simulink model "Controllers_Complete"  (R2021b)
settings: Solver=FixedStepAuto  StartTime=0  StopTime=20  FixedStep=0.002  RelTol=1e-3  EnableMultiTasking=on
PostLoadFcn:
  | qc_set_target_type(getConfigSet(bdroot, 'QUARC Default Target Configuration'));
values from neighbouring files (symbols this model uses):
  k = place(sysest_cont.A, sysest_cont.B, new_pole)    [Recursive.m]
  K_lqr = lqr(sysest_cont,Q,R)    [Recursive.m]
  K_p = 1/K_dc(1)    [AdaptivePPLvl2.m]
  K_pp = place(A, B, new_pole)    [AdaptivePPLvl2.m]
  Kr = 1/Kdc(1)    [Recursive.m]
  L_obs = place(sysest_cont.A',sysest_cont.C',1.5*new_pole)'    [Recursive.m]
  param = [disc(1).Numerator{:}(3:end) -disc(1).Denominator{:}(2:end)]    [Recursive.m]
  param2 = [disc(2).Numerator{:}(3:end) -disc(2).Denominator{:}(2:end)]    [Recursive.m]
  sysest_ct = sysest_cont    [Recursive.m]
  Trans = block.InputPort(1).Data    [AdaptivePPLvl2.m]
  Ts = 0.002    [AdaptivePPLvl2.m]
  v_a_max = 5    [Recursive.m]
undefined symbols (not defined in the file or in its folder): DiscIntNeverNeededParam, HIL, k2, K_lqr_eta, K_lqr_x, K_pp_en_eta, K_pp_en_x, Kr2, L22, L_KF, magnitude, Q_KF, qc_get_step_size, R_KF, sigbuilder_block, sysest, sysfake_ct
libraries: simulink_extras x7, ctrlSharedLib x4, quarc_library x4, cstblocks x1
settings Model: SimulationMode=external  ExtModeTrigDuration=5000  Creator=CFulford  LastModifiedBy=jesuc
settings SolverCC: AlgebraicLoopSolver=TrustRegion  PositivePriorityOrder=on
settings DataIOCC: LimitDataPoints=on  SaveFormat=Array  SignalLoggingSaveFormat=ModelDataLogs  ReturnWorkspaceOutputs=off
settings OptimizationCC: ExpressionDepthLimit=2147483647  InitFltsAndDblsToZero=on  LifeSpan=inf
settings DebuggingCC: SaveWithParameterizedLinksMsg=none  UnderspecifiedInitializationDetection=Classic  MergeDetectMultiDrivingBlocksExec=none  SolverPrmCheckMsg=warning  MultiTaskDSMMsg=warning  MultiTaskCondExecSysMsg=none  FcnCallInpInsideContextMsg=warning  StateNameClashWarn=warning  SFUnexpectedBacktrackingDiag=warning  SFNoUnconditionalDefaultTransitionDiag=warning  SFExecutionAtInitializationDiag=none  SFMachineParentedDataDiag=warning  ArithmeticOperatorsInVariantConditions=warning
settings HardwareCC: ProdBitPerPointer=32  ProdBitPerSizeT=32  ProdBitPerPtrDiffT=32  ProdLargestAtomicFloat=None  ProdIntDivRoundTo=Undefined  ProdEndianess=Unspecified  ProdWordSize=32  ProdHWDeviceType=32-bit Generic
settings ModelReferenceCC: PropagateSignalLabelsOutOfModel=off
settings SFSimCC: SimUseLocalCustomCode=off  CustomCodeUndefinedFunction=UseInterfaceOnly
settings RTWCC: Description=QUARC Win64 Target  SystemTargetFile=quarc_win64.tlc  TemplateMakefile=quarc_default_tmf  RTWUseLocalCustomCode=off
settings CodeAppCC: StateflowObjectComments=on
settings STFCustomTargetCC: TargetPreCompLibLocation=C:\PROGRA~3\QUARC\lib\2019b\win64\release  ConcurrentExecutionCompliant=on  CombineOutputUpdateFcns=on  CPPClassGenCompliant=on  GRTInterface=off  SystemTargetFile=quarc_win64.tlc
settings GRTTargetCC: TargetPreCompLibLocation=C:\PROGRA~3\QUARC\lib\2019b\win64\release  TargetLangStandard=C89/C90 (ANSI)  ParMdlRefBuildCompliant=off  CompOptLevelCompliant=off  MatFileLogging=off  UseToolchainInfoCompliant=off  ExtMode=on  ExtModeMexFile=quarc_comm
settings ConfigComp: CovMetricSettings=dw  CovSaveCumulativeToWorkspaceVar=on  CovSaveSingleToWorkspaceVar=on  CovExternalEMLEnable=off  CovSFcnEnable=off

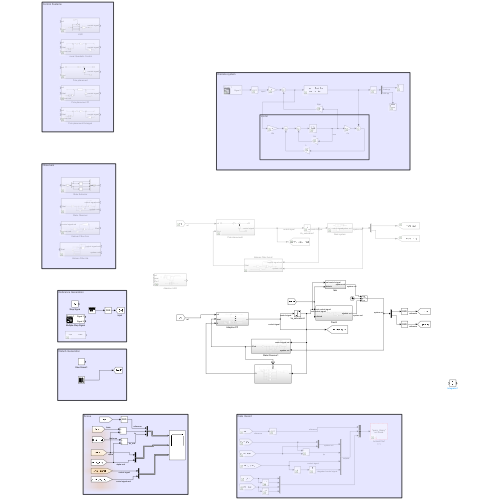
[thumbnail: Simulink's stored preview of the top-level diagram]
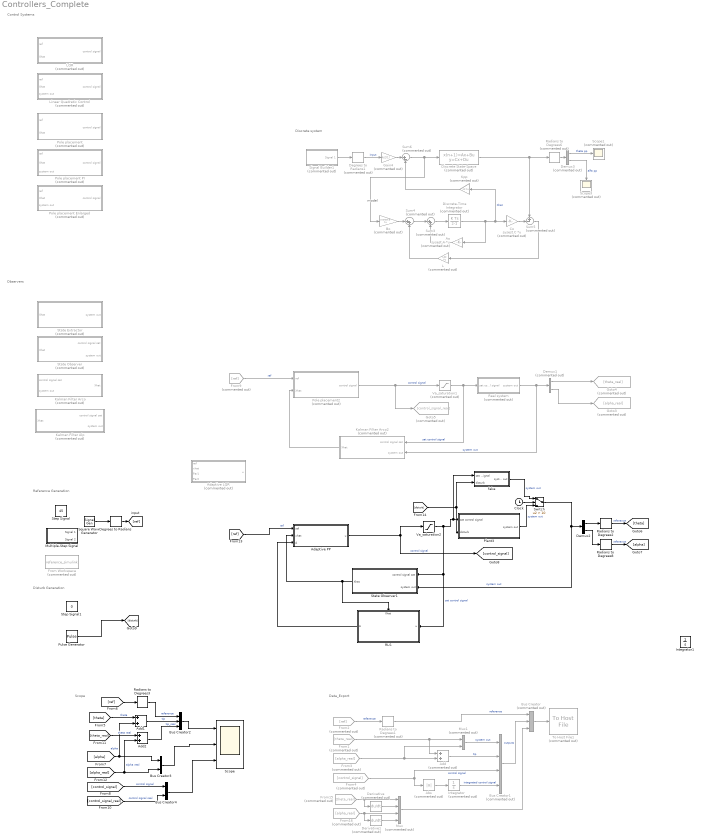
== system Controllers_Complete ==
  note: Reference Generation
  note: Disturb Generation
  note: Data_Export
  note: Scope
  note: Control Systems
  note: Observers
  note: Discrete system
  note: model
  Abs : Abs  Commented=on
  Adaptive LQR : Subsystem  Commented=on
  Adaptive PP : Subsystem
  Add : Sum  Commented=on
  Add1 : Sum
  Add2 : Sum
  Ao : Gain  Commented=on  Gain=sysest.A  Multiplication=Matrix(K*u)
  Bo : Gain  Commented=on  Gain=sysest.B  Multiplication=Matrix(K*u)
  Bus Creator : BusCreator  Commented=on  Inputs=3
  Bus Creator1 : BusCreator  Commented=on  Inputs=4
  Bus Creator2 : BusCreator  Inputs=3
  Bus Creator3 : BusCreator  Inputs=2
  Bus Creator4 : BusCreator  Inputs=2
  Clock : Clock
  Co : Gain  Commented=on  Gain=sysest.C  Multiplication=Matrix(K*u)
  Degrees to Radians : simulink_extras/Transformations/Degrees to Radians
  Degrees to Radians1 : simulink_extras/Transformations/Degrees to Radians  Commented=on
  Demux1 : Demux  Commented=on  Outputs=2
  Demux2 : Demux  Outputs=2
  Demux3 : Demux  Commented=on  Outputs=2
  Derivative : Derivative  Commented=on
  Derivative1 : Derivative  Commented=on
  Discrete State-Space : DiscreteStateSpace  Commented=on  A=sysest.A  B=sysest.B  C=sysest.C  D=sysest.D  SampleTime=0.002
  Discrete-Time Integrator : DiscreteIntegrator  Commented=on  SampleTime=0.002  ICPrevOutput=DiscIntNeverNeededParam  ICPrevScaledInput=DiscIntNeverNeededParam
  From Workspace : FromWorkspace  Commented=on  VariableName=reference_simulink
  From1 : From  Commented=on  GotoTag=theta_real
  From15 : From  Commented=on  GotoTag=theta_real
  From16 : From  Commented=on  GotoTag=alpha_real
  From2 : From  Commented=on  GotoTag=ref
  From3 : From  Commented=on  GotoTag=alpha_real
  From4 : From  Commented=on  GotoTag=control_signal
  From9 : From  Commented=on  GotoTag=ref
  Gain4 : Gain  Commented=on  Gain=Kr2(1)
  Goto3 : Goto  Commented=on  GotoTag=alpha_real
  Goto4 : Goto  Commented=on  GotoTag=theta_real
  Goto5 : Goto  Commented=on  GotoTag=control_signal_real
  Integrator : Integrator  Commented=on
  Integrator1 : Integrator
  Kalman Filter Alp : Subsystem  Commented=on
  Kalman Filter Arco : Subsystem  Commented=on
  Kalman Filter Arco2 : Subsystem  Commented=on
  Kpp : Gain  Commented=on  Gain=k2  Multiplication=Matrix(K*u)
  L : Gain  Commented=on  Gain=L22  Multiplication=Matrix(K*u)
  LQR : Subsystem  Commented=on
  Linear Quadratic Control : Subsystem  Commented=on
  Multiple-Step Signal : Subsystem  Tag=STV Subsys  LoadFcn=sigbuilder_block('load');  StartFcn=sigbuilder_block('start');  StopFcn=sigbuilder_block('stop');  ClipboardFcn=sigbuilder_block('clipboard');  mask(Sigbuilder block){tuvar=[0:10]}
      mask help: Simulink:masks:SigbuilderBlock_MD
      mask init:
      | if ~strcmp(get_param(bdroot(gcbh),'SimulationStatus'),'stopped') tuvar = sigbuilder_block('maskInit'); end
      settings: CopyFcn=sigbuilder_block('copy');  DeleteFcn=sigbuilder_block('delete');  ModelCloseFcn=sigbuilder_block('modelClose');  PreSaveFcn=sigbuilder_block('preSave');  PauseFcn=sigbuilder_block('pause');  ContinueFcn=sigbuilder_block('continue');  NameChangeFcn=sigbuilder_block('namechange');  OpenFcn=sigbuilder_block('open',[5.4 5.4 1141.2 580.8 ]);  CloseFcn=sigbuilder_block('close');
      mask Display: plot(0, 0, 100, 100,[2, 2, 32, 32, 2], [68, 8, 8, 68, 68],[32, 2], [38, 38], [32, 19, 2],[53, 60, 44], [32, 17, 17, 2],[16, 16, 31, 31]);txt = getActiveGroup(gcbh);text(2, 100, txt,'verticalAlignment', 'top');
  Mux : Mux  Commented=on
  Mux1 : Mux  Commented=on  Inputs=2
  Plant3 : Subsystem
  Pole placement : Subsystem  Commented=on
  Pole placement Enlarged : Subsystem  Commented=on
  Pole placement PI : Subsystem  Commented=on
  Pole placement2 : Subsystem  Commented=on
  Pulse Generator : DiscretePulseGenerator  PulseType=Time based  Amplitude=0.001  Period=1  PulseWidth=50
  RLS : Subsystem
      settings: PortSchema="{\"entries\":[{\"content\":{\"sides\":[{\"content\":{\"connectorIds\":[\"In1\"]},\"type\":\"ConnectorPlacement.EquallySpacedRectSide\",\"uuid\":\"553c4a9d-f21a-4a66-a87a-a243cd55d2e3\"},{\"content\":{\"connectorIds\":[\"Out1\"],\"side\":\"RIGHT\"},\"type\":\"ConnectorPlacement.EquallySpacedRectSide\",\"uuid\":\"7c0c7ce9-5483-43cc-b177-6c3304c50a8e\"},{\"content\":{\"connectorIds\":[\"In2\"],\"side\":\"TOP\"},\"type\":\"ConnectorPlacement.EquallySpacedRectSide\",\"uuid\":\"5face929-888d-4c99-9f40-f5add7f5ece6\"}]},\"type\":\"ConnectorPlacement.EquallySpacedConnector\",\"uuid\":\"9b2ed38d-f553-46ca-b742-367219c23a2d\"}],\"packageUris\":[\"http://schema.mathworks.com/mf0/Connector/R2020b\"],\"version\":\"1.0\"}"
  Radians to Degrees1 : simulink_extras/Transformations/Radians to Degrees  Commented=on
  Radians to Degrees2 : simulink_extras/Transformations/Radians to Degrees
  Radians to Degrees3 : simulink_extras/Transformations/Radians to Degrees
  Radians to Degrees6 : simulink_extras/Transformations/Radians to Degrees  Commented=on
  Radians to Degrees8 : simulink_extras/Transformations/Radians to Degrees
  Real system : Subsystem  Commented=on
  Scope : Scope  NumInputPorts=3
  Scope1 : Scope  Commented=on
  Scope3 : Scope  Commented=on
  Signal Builder1 : Subsystem  Tag=STV Subsys  Commented=on  LoadFcn=sigbuilder_block('load');  StartFcn=sigbuilder_block('start');  StopFcn=sigbuilder_block('stop');  ClipboardFcn=sigbuilder_block('clipboard');  mask(Sigbuilder block){tuvar=[0:10]}
      mask help: Simulink:masks:SigbuilderBlock_MD
      mask init:
      | if ~strcmp(get_param(bdroot(gcbh),'SimulationStatus'),'stopped') tuvar = sigbuilder_block('maskInit'); end
      settings: CopyFcn=sigbuilder_block('copy');  DeleteFcn=sigbuilder_block('delete');  ModelCloseFcn=sigbuilder_block('modelClose');  PreSaveFcn=sigbuilder_block('preSave');  PauseFcn=sigbuilder_block('pause');  ContinueFcn=sigbuilder_block('continue');  NameChangeFcn=sigbuilder_block('namechange');  OpenFcn=sigbuilder_block('open',[437.6 199.2 550.4 400 ]);  CloseFcn=sigbuilder_block('close');
      mask Display: plot(0, 0, 100, 100,[2, 2, 32, 32, 2], [68, 8, 8, 68, 68],[32, 2], [38, 38], [32, 19, 2],[53, 60, 44], [32, 17, 17, 2],[16, 16, 31, 31]);txt = getActiveGroup(gcbh);text(2, 100, txt,'verticalAlignment', 'top');
  Square Wave Generator : SignalGenerator  WaveForm=square  Amplitude=45  Frequency=3  Units=rad/sec
  State Extractor : Subsystem  Commented=on
  State Observer : Subsystem  Commented=on
  State Observer1 : Subsystem
  Step Signal : Constant  Value=45
  Step Signal1 : Constant  Value=0
  Sum3 : Sum  Commented=on  Inputs=|++
  Sum4 : Sum  Commented=on  Inputs=|++
  Sum5 : Sum  Commented=on  Inputs=+-|
  Sum6 : Sum  Commented=on  Inputs=|+-
  Switch : Switch  Criteria=u2 > Threshold  Threshold=10
  To Host File1 : quarc_library/Sinks/To Host/To Host File  Commented=on  file_name=Sine tests\Sine_24_in_theta_alpha.mat  variable_name=data  decimation=1  sample_time=-1  file_format=MAT-file v.4  options=No header or footer  append=off  final_file_name=Sine tests\Sine_24_in_theta_alpha.mat  bitrate=2000000
  Va_saturation1 : Saturate  Commented=on  UpperLimit=v_a_max  LowerLimit=-v_a_max
  Va_saturation2 : Saturate  UpperLimit=v_a_max  LowerLimit=-v_a_max
  fake : Subsystem
  wires:
  Bus Creator2/1 -> Scope/1
  Bus Creator3/1 -> Scope/2
  Pole placement2/1(" control signal") -> Goto5/1, Va_saturation1/1  "control signal"
  From4/1 -> Abs/1, Bus Creator1/3  "control signal"
  Bus Creator1/1 -> Bus Creator/2  "outputs"
  [disturb] -> fake/2(disturb), Plant3/2(disturb)
  Demux2/1 -> Radians to Degrees2/1
  Adaptive PP/1(u) -> Va_saturation2/1, [control_signal]  "control signal"
  [ref] -> Adaptive PP/1(ref)  "ref"
  From1/1 -> Add/1, Mux1/1
  [control_signal_real] -> Bus Creator4/2  "control signal real"
  Add/1 -> Bus Creator1/2  "tip"
  From2/1 -> Radians to Degrees1/1  "reference"
  Integrator/1 -> Bus Creator1/4  "integrated control signal"
  Bus Creator/1 -> To Host File1/1
  [alpha_real] -> Bus Creator3/2, Add2/2  "alpha real"
  Demux1/1 -> Goto4/1
  Real system/1(system out) -> Kalman Filter Arco2/2(system out), Demux1/1  "system out"
  [theta_real] -> Add2/1  "theta real"
  Va_saturation2/1 -> State Observer1/1(control signal sat), RLS/1(u), Plant3/1(sat control signal), fake/1(sat control signal)  "sat control signal"
  From3/1 -> Add/2, Mux1/2
  Demux1/2 -> Goto3/1
  Switch/1 -> State Observer1/2(system out), Demux2/1  "system out"
  [control_signal] -> Bus Creator4/1  "control signal"
  Degrees to Radians/1 -> [ref]
  Bus Creator4/1 -> Scope/3
  Radians to Degrees3/1 -> Bus Creator2/1  "reference"
  Va_saturation1/1 -> Kalman Filter Arco2/1(control signal sat), Real system/1(sat control signal)  "sat control signal"
  [alpha] -> Bus Creator3/1, Add1/2  "alpha"
  Mux1/1 -> Bus Creator1/1  "system out"
  [theta] -> Add1/1  "theta"
  Demux2/2 -> Radians to Degrees8/1
  Sum5/1 -> L/1
  Demux3/1 -> Scope1/1  "theta pp"
  Sum6/1 -> Discrete State-Space/1, Bo/1
  L/1 -> Sum4/2
  Discrete State-Space/1 -> Radians to Degrees6/1, Sum5/1
  Sum4/1 -> Sum3/1
  Sum3/1 -> Discrete-Time Integrator/1
  Degrees to Radians1/1 -> Gain4/1  "input"
  Co/1 -> Sum5/2
  Demux3/2 -> Scope3/1  "alfa pp"
  Signal Builder1/1(Signal 1) -> Degrees to Radians1/1
  Kpp/1 -> Sum6/2
  Bo/1 -> Sum4/1
  Discrete-Time Integrator/1 -> Ao/1, Kpp/1, Co/1  "Xhat"
  Gain4/1 -> Sum6/1
  Ao/1 -> Sum3/2
  Radians to Degrees6/1 -> Demux3/1
  From9/1 -> Pole placement2/1(ref)  "ref"
  Add1/1 -> Bus Creator2/2  "tip"
  Add2/1 -> Bus Creator2/3  "tip_real"
  [ref] -> Radians to Degrees3/1
  Radians to Degrees1/1 -> Bus Creator/1  "reference"
  Radians to Degrees2/1 -> [theta]  "reference"
  Radians to Degrees8/1 -> [alpha]  "reference"
  State Observer1/1(Xhat) -> Adaptive PP/2(xhat), RLS/2(Xhat)
  Kalman Filter Arco2/1(Xhat) -> Pole placement2/2(Xhat)
  Abs/1 -> Integrator/1
  From15/1 -> Derivative/1, Mux/1
  From16/1 -> Derivative1/1, Mux/3
  Mux/1 -> Bus Creator/3
  Derivative/1 -> Mux/2
  Derivative1/1 -> Mux/4
  RLS/1(A) -> Adaptive PP/3(A)
  Pulse Generator/1 -> [disturb]
  fake/1(system out) -> Switch/1  "system out"
  Plant3/1(system out) -> Switch/3  "system out"
  Square Wave Generator/1 -> Degrees to Radians/1
  Clock/1 -> Switch/2

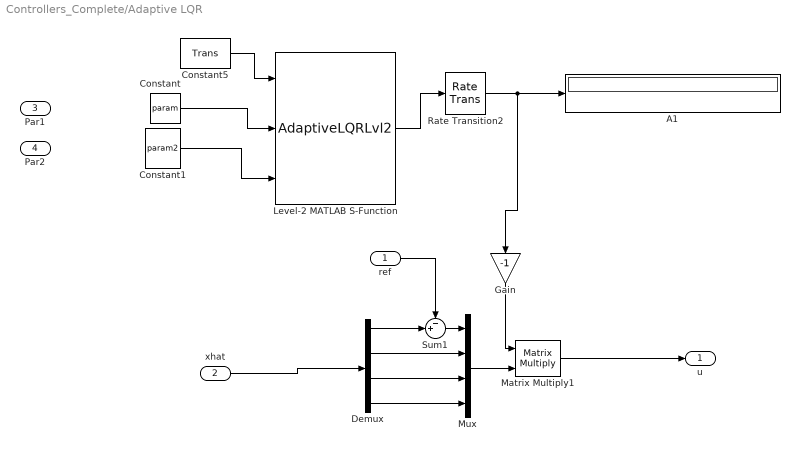
== system Controllers_Complete/Adaptive LQR ==
  ref : Inport
  xhat : Inport  Port=2
  Par1 : Inport  Port=3
  Par2 : Inport  Port=4
  A1 : Display
  Constant : Constant  Value=param
  Constant1 : Constant  Value=param2
  Constant5 : Constant  Value=Trans  SampleTime=Ts
  Demux : Demux
  Gain : Gain  Gain=-1
  Level-2 MATLAB S-Function : M-S-Function  FunctionName=AdaptiveLQRLvl2
  Matrix Multiply1 : Product  Multiplication=Matrix(*)
  Mux : Mux
  Rate Transition2 : RateTransition  InitialCondition=k
  Sum1 : Sum  Inputs=-+|
  u : Outport
  wires:
  Constant5/1 -> Level-2 MATLAB S-Function/1
  Constant/1 -> Level-2 MATLAB S-Function/2
  Level-2 MATLAB S-Function/1 -> Rate Transition2/1
  Rate Transition2/1 -> Gain/1, A1/1
  Constant1/1 -> Level-2 MATLAB S-Function/3
  ref/1 -> Sum1/1
  Sum1/1 -> Mux/1
  Demux/2 -> Mux/2
  Demux/4 -> Mux/4
  Demux/3 -> Mux/3
  Demux/1 -> Sum1/2
  xhat/1 -> Demux/1
  Matrix Multiply1/1 -> u/1
  Mux/1 -> Matrix Multiply1/2
  Gain/1 -> Matrix Multiply1/1

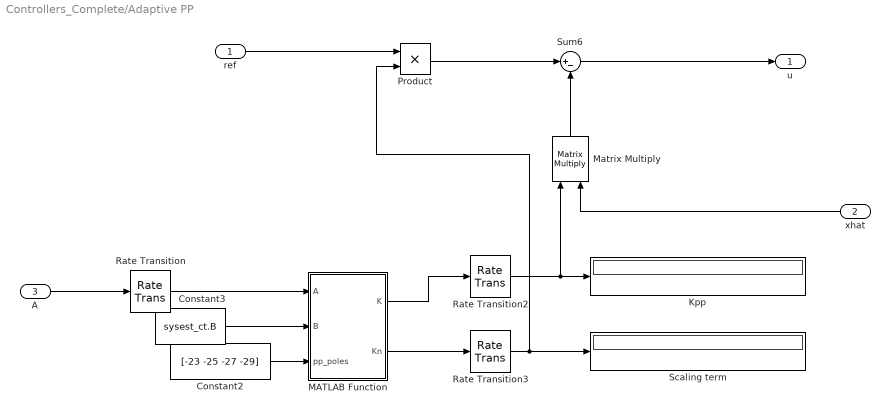
== system Controllers_Complete/Adaptive PP ==
  ref : Inport
  xhat : Inport  Port=2
  A : Inport  Port=3
  Constant2 : Constant  Value=[-23 -25 -27 -29]  SampleTime=0.2
  Constant3 : Constant  Value=sysest_ct.B  SampleTime=0.2
  Kpp : Display
  MATLAB Function : MATLAB Function  TreatAsAtomicUnit=on
  Matrix Multiply : Product  Multiplication=Matrix(*)
  Product : Product
  Rate Transition : RateTransition  InitialCondition=sysest_ct.A  OutPortSampleTime=0.2
  Rate Transition2 : RateTransition  InitialCondition=k
  Rate Transition3 : RateTransition  InitialCondition=Kr
  Scaling term : Display
  Sum6 : Sum  Inputs=|+-
  u : Outport
  wires:
  Product/1 -> Sum6/1
  Sum6/1 -> u/1
  Matrix Multiply/1 -> Sum6/2
  ref/1 -> Product/1
  MATLAB Function/2(Kn) -> Rate Transition3/1
  Rate Transition/1 -> MATLAB Function/1(A)
  MATLAB Function/1(K) -> Rate Transition2/1
  Rate Transition2/1 -> Kpp/1, Matrix Multiply/1
  Rate Transition3/1 -> Product/2, Scaling term/1
  xhat/1 -> Matrix Multiply/2
  A/1 -> Rate Transition/1
  Constant2/1 -> MATLAB Function/3(pp_poles)
  Constant3/1 -> MATLAB Function/2(B)

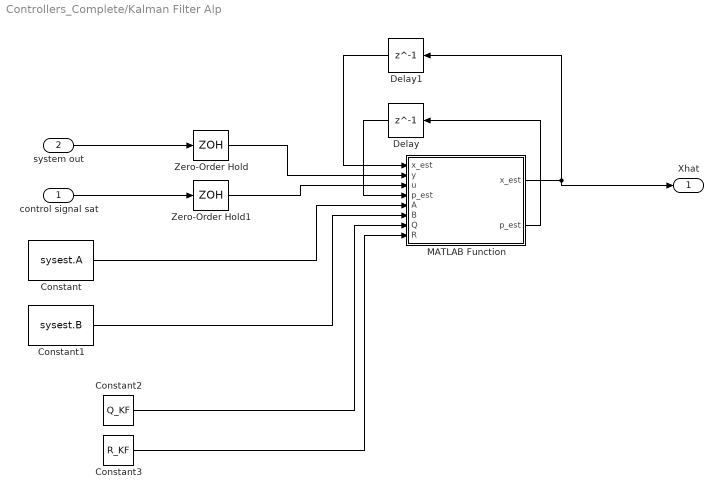
== system Controllers_Complete/Kalman Filter Alp ==
  control signal sat : Inport
  system out : Inport  Port=2
  Constant : Constant  Value=sysest.A
  Constant1 : Constant  Value=sysest.B
  Constant2 : Constant  Value=Q_KF
  Constant3 : Constant  Value=R_KF
  Delay : Delay  DelayLength=1  InitialCondition=eye(4)
  Delay1 : Delay  DelayLength=1  InitialCondition=[0;0;0;0]
  MATLAB Function : MATLAB Function  TreatAsAtomicUnit=on
  Zero-Order Hold : ZeroOrderHold  SampleTime=0.002
  Zero-Order Hold1 : ZeroOrderHold  SampleTime=0.002
  Xhat : Outport
  wires:
  MATLAB Function/1(x_est) -> Xhat/1, Delay1/1
  Delay/1 -> MATLAB Function/4("p_est ")
  MATLAB Function/2(p_est) -> Delay/1
  Zero-Order Hold1/1 -> MATLAB Function/3(u)
  Constant1/1 -> MATLAB Function/6(B)
  Delay1/1 -> MATLAB Function/1("x_est ")
  Constant/1 -> MATLAB Function/5(A)
  Zero-Order Hold/1 -> MATLAB Function/2(y)
  control signal sat/1 -> Zero-Order Hold1/1
  system out/1 -> Zero-Order Hold/1
  Constant2/1 -> MATLAB Function/7(Q)
  Constant3/1 -> MATLAB Function/8(R)

== system Controllers_Complete/Kalman Filter Arco ==
  control signal sat : Inport  PortDimensions=1
  system out : Inport  Port=2  PortDimensions=2
  Add : Sum  Inputs=+++
  Gain : Gain  Gain=sysest_ct.B  Multiplication=Matrix(K*u) (u vector)
  Gain1 : Gain  Gain=L_KF  Multiplication=Matrix(K*u) (u vector)
  Gain2 : Gain  Gain=sysest_ct.A - L_KF * sysest_ct.C  Multiplication=Matrix(K*u) (u vector)
  Integrator : Integrator
  Xhat : Outport  PortDimensions=4
  wires:
  Gain2/1 -> Add/1
  Integrator/1 -> Gain2/1, Xhat/1  "x_hat"
  Add/1 -> Integrator/1  "x_hat_dot"
  Gain/1 -> Add/2
  control signal sat/1 -> Gain/1
  Gain1/1 -> Add/3
  system out/1 -> Gain1/1

== system Controllers_Complete/Kalman Filter Arco2 ==
  control signal sat : Inport  PortDimensions=1
  system out : Inport  Port=2  PortDimensions=2
  Add : Sum  Inputs=+++
  Gain : Gain  Gain=sysest_ct.B  Multiplication=Matrix(K*u) (u vector)
  Gain1 : Gain  Gain=L_KF  Multiplication=Matrix(K*u) (u vector)
  Gain2 : Gain  Gain=sysest_ct.A - L_KF * sysest_ct.C  Multiplication=Matrix(K*u) (u vector)
  Integrator : Integrator
  Xhat : Outport  PortDimensions=4
  wires:
  Gain2/1 -> Add/1
  Integrator/1 -> Gain2/1, Xhat/1  "x_hat"
  Add/1 -> Integrator/1  "x_hat_dot"
  Gain/1 -> Add/2
  control signal sat/1 -> Gain/1
  Gain1/1 -> Add/3
  system out/1 -> Gain1/1

== system Controllers_Complete/LQR ==
  ref : Inport
  Xhat : Inport  Port=2
  Demux : Demux
  Gain3 : Gain  Gain=-K_lqr  Multiplication=Matrix(K*u)
  Mux : Mux
  Sum1 : Sum  Inputs=-+|
  " control signal" : Outport
  wires:
  ref/1 -> Sum1/1
  Xhat/1 -> Demux/1
  Demux/1 -> Sum1/2
  Demux/2 -> Mux/2
  Demux/3 -> Mux/3
  Demux/4 -> Mux/4
  Gain3/1 -> " control signal"/1
  Sum1/1 -> Mux/1
  Mux/1 -> Gain3/1

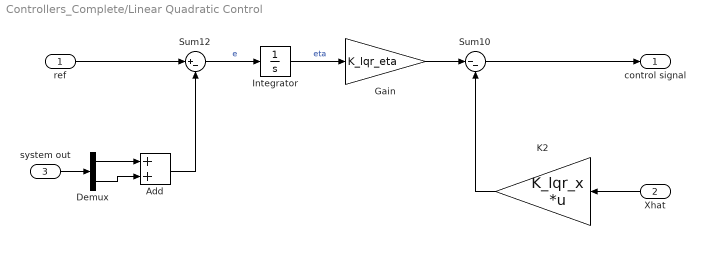
== system Controllers_Complete/Linear Quadratic Control ==
  ref : Inport
  Xhat : Inport  Port=2
  system out : Inport  Port=3
  Add : Sum
  Demux : Demux  Outputs=2
  Gain : Gain  Gain=K_lqr_eta
  Integrator : Integrator
  K2 : Gain  Gain=K_lqr_x  Multiplication=Matrix(K*u)
  Sum10 : Sum  Inputs=|--
  Sum12 : Sum  Inputs=|+-
  " control signal" : Outport
  wires:
  ref/1 -> Sum12/1
  Gain/1 -> Sum10/1
  Integrator/1 -> Gain/1  "eta"
  Sum10/1 -> " control signal"/1
  K2/1 -> Sum10/2
  Add/1 -> Sum12/2
  Sum12/1 -> Integrator/1  "e"
  Xhat/1 -> K2/1
  system out/1 -> Demux/1
  Demux/2 -> Add/2
  Demux/1 -> Add/1

== system Controllers_Complete/Multiple-Step Signal ==
  Demux : Demux  Tag=STV Demux  Outputs=2
      settings: DisplayOption=none
  FromWs : FromWorkspace  Tag=STV FromWs  VariableName=tuvar
      SigBuilderData=|
      | common.afterFinalStr = 'Extrapolate'
      | common.sampleTime = 0
      | dataSet.timeRange = [0 10]
      | dataSet.name = 'Group 1'
      | sbobj.Groups.Name = 'Group 1'
      | sbobj.Groups.Signals(1).Name = 'Signal 1'
      | sbobj.Groups.Signals(1).XData = [0 1 1 3 3 7 7 8.5 8.5 10]
      | sbobj.Groups.Signals(1).YData = [0.005 0.005 40 40 -30 -30 0 0 23 23]
      | sbobj.Groups.Signals(2).Name = 'Signal 2'
      | sbobj.Groups.Signals(2).XData = [0 1 1 1.52 10]
      | sbobj.Groups.Signals(2).YData = [0 0 -40 -40 -40]
  Signal 1 : Outport  Tag=STV Outport
  Signal 2 : Outport  Tag=STV Outport  Port=2
  wires:
  Demux/1 -> Signal 1/1
  FromWs/1 -> Demux/1
  Demux/2 -> Signal 2/1

== system Controllers_Complete/Plant3 ==
  sat control signal : Inport
  disturb : Inport  Port=2
  A1 : Gain  Gain=sysest_ct.A  Multiplication=Matrix(K*u)
  B1 : Gain  Gain=sysest_ct.B  Multiplication=Matrix(K*u)
  C1 : Gain  Gain=sysest_ct.C  Multiplication=Matrix(K*u)
  Integrator2 : Integrator
  Sum7 : Sum  Inputs=|++
  Sum9 : Sum  Inputs=++|
  system out : Outport
  wires:
  Sum7/1 -> Integrator2/1
  disturb/1 -> Sum9/1
  B1/1 -> Sum7/1
  Integrator2/1 -> A1/1, C1/1  "xhat"
  C1/1 -> system out/1  "y"
  A1/1 -> Sum7/2
  sat control signal/1 -> Sum9/2
  Sum9/1 -> B1/1

== system Controllers_Complete/Pole placement ==
  ref : Inport
  Xhat : Inport  Port=2
  Gain4 : Gain  Gain=K_p
  K : Gain  Gain=K_pp  Multiplication=Matrix(K*u)
  Sum1 : Sum  Inputs=|+-
  " control signal" : Outport
  wires:
  K/1 -> Sum1/2
  Xhat/1 -> K/1
  Sum1/1 -> " control signal"/1  "u"
  Gain4/1 -> Sum1/1
  ref/1 -> Gain4/1

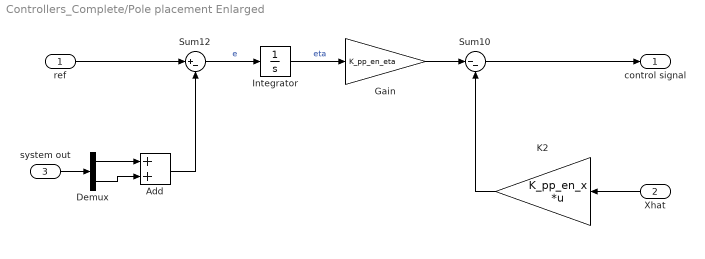
== system Controllers_Complete/Pole placement Enlarged ==
  ref : Inport
  Xhat : Inport  Port=2
  system out : Inport  Port=3
  Add : Sum
  Demux : Demux  Outputs=2
  Gain : Gain  Gain=K_pp_en_eta
  Integrator : Integrator
  K2 : Gain  Gain=K_pp_en_x  Multiplication=Matrix(K*u)
  Sum10 : Sum  Inputs=|--
  Sum12 : Sum  Inputs=|+-
  " control signal" : Outport
  wires:
  ref/1 -> Sum12/1
  Gain/1 -> Sum10/1
  Integrator/1 -> Gain/1  "eta"
  Sum10/1 -> " control signal"/1
  K2/1 -> Sum10/2
  Add/1 -> Sum12/2
  Sum12/1 -> Integrator/1  "e"
  Xhat/1 -> K2/1
  system out/1 -> Demux/1
  Demux/2 -> Add/2
  Demux/1 -> Add/1

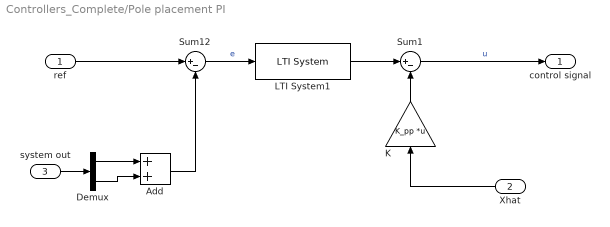
== system Controllers_Complete/Pole placement PI ==
  ref : Inport
  Xhat : Inport  Port=2
  system out : Inport  Port=3
  Add : Sum
  Demux : Demux  Outputs=2
  K : Gain  Gain=K_pp  Multiplication=Matrix(K*u)
  LTI System1 : cstblocks/LTI System  sys=PI_pp  IC=[]
  Sum1 : Sum  Inputs=|+-
  Sum12 : Sum  Inputs=|+-
  " control signal" : Outport
  wires:
  K/1 -> Sum1/2
  Xhat/1 -> K/1
  Sum1/1 -> " control signal"/1  "u"
  LTI System1/1 -> Sum1/1
  Sum12/1 -> LTI System1/1  "e"
  Demux/1 -> Add/1
  system out/1 -> Demux/1
  Add/1 -> Sum12/2
  Demux/2 -> Add/2
  ref/1 -> Sum12/1

== system Controllers_Complete/Pole placement2 ==
  ref : Inport
  Xhat : Inport  Port=2
  Gain4 : Gain  Gain=K_p
  K : Gain  Gain=K_pp  Multiplication=Matrix(K*u)
  Sum1 : Sum  Inputs=|+-
  " control signal" : Outport
  wires:
  K/1 -> Sum1/2
  Xhat/1 -> K/1
  Sum1/1 -> " control signal"/1  "u"
  Gain4/1 -> Sum1/1
  ref/1 -> Gain4/1

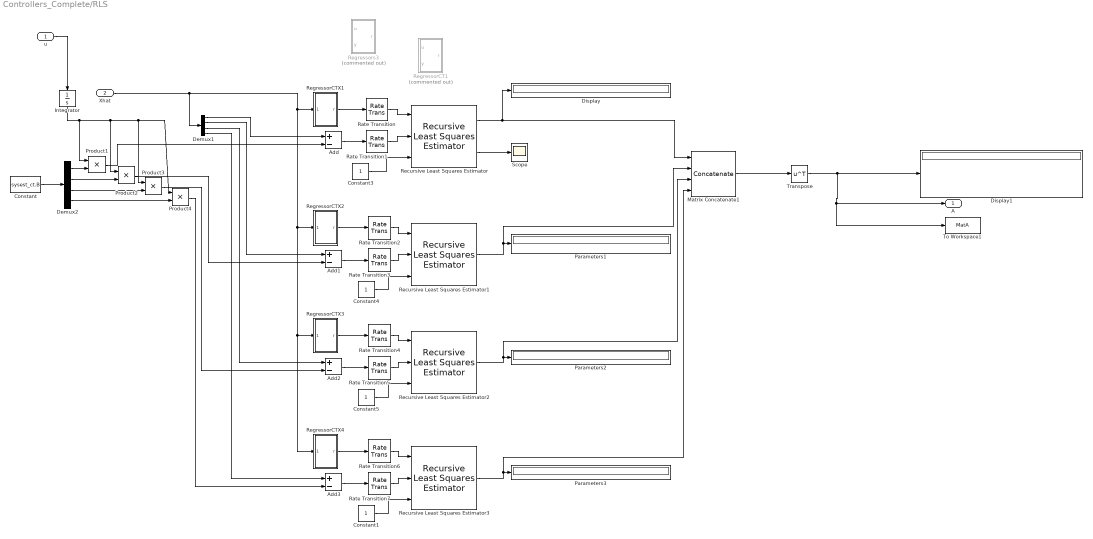
== system Controllers_Complete/RLS ==
  u : Inport
  Xhat : Inport  Port=2
  Add{,1..3} (4 alike) : Sum  Inputs=+-
  Constant : Constant  Value=sysest_ct.B
  Constant{1,3..5} (4 alike) : Constant  SampleTime=0.002
  Demux1 : Demux
  Demux2 : Demux
  Display : Display
  Display1 : Display
  Integrator : Integrator
  Matrix Concatenate1 : Concatenate  NumInputs=4  Mode=Multidimensional array  ConcatenateDimension=2
  Parameters1 : Display
  Parameters2 : Display
  Parameters3 : Display
  Product{1..4} (4 alike) : Product
  Rate Transition{,1..7} (8 alike) : RateTransition  OutPortSampleTime=0.002
  Recursive Least Squares Estimator : ctrlSharedLib/Recursive Least Squares Estimator  InitialEstimateSource=Internal  InitialParameterData=[ 0 1 -0.6 -0.0001]  P0=10  InitialRegressors=0  InitialOutputs=0  History=Infinite  WindowLength=100  EstimationMethod=Forgetting Factor  AdaptationParameter=1-1e-4  HasTimeVaryingAdaptationParameter=off  NormalizationBias=eps  OutputError=on  OutputP=off  AddEnablePort=off  ExternalReset=Falling  InputProcessing=Sample-based  Ts=0.002
      settings: SourceProductBaseCode=CT,ID
  Recursive Least Squares Estimator1 : ctrlSharedLib/Recursive Least Squares Estimator  InitialEstimateSource=Internal  InitialParameterData=[0 -37 600 0.27]  P0=10  InitialRegressors=0  InitialOutputs=0  History=Infinite  WindowLength=100  EstimationMethod=Forgetting Factor  AdaptationParameter=1-1e-4  HasTimeVaryingAdaptationParameter=off  NormalizationBias=eps  OutputError=off  OutputP=off  AddEnablePort=off  ExternalReset=Falling  InputProcessing=Sample-based  Ts=0.002
      settings: SourceProductBaseCode=CT,ID
  Recursive Least Squares Estimator2 : ctrlSharedLib/Recursive Least Squares Estimator  InitialEstimateSource=Internal  InitialParameterData=[0 -0.0377 0.9948 1.0002]  P0=10  InitialRegressors=0  InitialOutputs=0  History=Infinite  WindowLength=100  EstimationMethod=Forgetting Factor  AdaptationParameter=1-1e-4  HasTimeVaryingAdaptationParameter=off  NormalizationBias=eps  OutputError=off  OutputP=off  AddEnablePort=off  ExternalReset=Falling  InputProcessing=Sample-based  Ts=0.002
      settings: SourceProductBaseCode=CT,ID
  Recursive Least Squares Estimator3 : ctrlSharedLib/Recursive Least Squares Estimator  InitialEstimateSource=Internal  InitialParameterData=[0 37.2 -987.4 -0.45]  P0=10  InitialRegressors=0  InitialOutputs=0  History=Infinite  WindowLength=100  EstimationMethod=Forgetting Factor  AdaptationParameter=1-1e-4  HasTimeVaryingAdaptationParameter=off  NormalizationBias=eps  OutputError=off  OutputP=off  AddEnablePort=off  ExternalReset=Falling  InputProcessing=Sample-based  Ts=0.002
      settings: SourceProductBaseCode=CT,ID
  RegressorCT1 : Subsystem  Commented=on
  RegressorCTX1 : Subsystem
  RegressorCTX2 : Subsystem
  RegressorCTX3 : Subsystem
  RegressorCTX4 : Subsystem
  Regressors3 : Subsystem  Commented=on
  Scope : Scope
  To Workspace1 : ToWorkspace  VariableName=MatA  SaveFormat=Timeseries  SampleTime=0.002
  Transpose : Math  Operator=transpose  SaturateOnIntegerOverflow=on
  A : Outport
  wires:
  Recursive Least Squares Estimator/2 -> Scope/1
  Rate Transition2/1 -> Recursive Least Squares Estimator1/1
  Rate Transition3/1 -> Recursive Least Squares Estimator1/2
  RegressorCTX2/1(r) -> Rate Transition2/1
  RegressorCTX1/1(r) -> Rate Transition/1
  Rate Transition/1 -> Recursive Least Squares Estimator/1
  Rate Transition1/1 -> Recursive Least Squares Estimator/2
  Xhat/1 -> RegressorCTX4/1(Xhat), RegressorCTX3/1(Xhat), RegressorCTX2/1(Xhat), RegressorCTX1/1(Xhat), Demux1/1
  Demux2/1 -> Product1/2
  Product1/1 -> Add/2
  Add/1 -> Rate Transition1/1
  Constant/1 -> Demux2/1
  Demux1/1 -> Add/1
  u/1 -> Integrator/1
  Demux1/2 -> Add1/1
  Demux2/2 -> Product2/2
  Product2/1 -> Add1/2
  Add1/1 -> Rate Transition3/1
  Recursive Least Squares Estimator1/1 -> Matrix Concatenate1/2, Parameters1/1
  Recursive Least Squares Estimator/1 -> Display/1, Matrix Concatenate1/1
  Matrix Concatenate1/1 -> Transpose/1
  Constant3/1 -> Recursive Least Squares Estimator/3
  Constant4/1 -> Recursive Least Squares Estimator1/3
  Rate Transition4/1 -> Recursive Least Squares Estimator2/1
  RegressorCTX3/1(r) -> Rate Transition4/1
  Constant5/1 -> Recursive Least Squares Estimator2/3
  Rate Transition5/1 -> Recursive Least Squares Estimator2/2
  Add2/1 -> Rate Transition5/1
  Demux2/3 -> Product3/2
  Product3/1 -> Add2/2
  Demux1/3 -> Add2/1
  Recursive Least Squares Estimator2/1 -> Matrix Concatenate1/3, Parameters2/1
  Integrator/1 -> Product4/1, Product3/1, Product2/1, Product1/1
  Recursive Least Squares Estimator3/1 -> Matrix Concatenate1/4, Parameters3/1
  Product4/1 -> Add3/2
  Demux1/4 -> Add3/1
  RegressorCTX4/1(r) -> Rate Transition6/1
  Rate Transition7/1 -> Recursive Least Squares Estimator3/2
  Rate Transition6/1 -> Recursive Least Squares Estimator3/1
  Constant1/1 -> Recursive Least Squares Estimator3/3
  Add3/1 -> Rate Transition7/1
  Demux2/4 -> Product4/2
  Transpose/1 -> A/1, To Workspace1/1, Display1/1

== system Controllers_Complete/Real system ==
  sat control signal : Inport
  Encoders : quarc_library/Data Acquisition/Generic/Timebases/HIL Read Encoder Timebase  object_name=HIL-1  clock=0  channels=[0:1]  samples_in_buffer=max(ceil(1/qc_get_step_size), 1)  active=on  vector_output=off  data_type_mode=Inherit via back propagation  data_type=double
  Gain : Gain  Gain=-1
  HIL Initialize : quarc_library/Data Acquisition/Generic/Configuration/HIL Initialize  Priority=-99  object_name=HIL-1  board_type=q2_usb  board_number=0  board_options=d0=digital;d1=digital;led=auto;update_rate=normal;decimation=1  exclusive=off  active=off  hardware_clocks=[0]  clock_modes=[]  initial_clock_frequencies=[]  set_clock_params_at_start=off  set_clock_params_at_switch_in=off  set_clock_frequencies_at_start=off  set_clock_frequencies_at_switch_in=off  analog_input_channels=[0:1]  analog_input_configurations=[]  analog_input_maximums=10  analog_input_minimums=-10  set_analog_input_params_at_start=on  set_analog_input_params_at_switch_in=off  analog_output_channels=[0:1]  analog_output_maximums=10  analog_output_minimums=-10  initial_analog_outputs=[0]  final_analog_outputs=[0]  watchdog_analog_outputs=0  set_analog_output_params_at_start=on  set_analog_output_params_at_switch_in=off  set_analog_outputs_at_start=on  set_analog_outputs_at_switch_in=off  set_analog_outputs_at_terminate=on  set_analog_outputs_at_switch_out=off  set_analog_outputs_on_watchdog=off  digital_input_channels=[]  digital_output_channels=[]  digital_output_configuration=[]  initial_digital_outputs=[1]  final_digital_outputs=[1]  watchdog_digital_outputs=[1]  set_digital_output_params_at_start=off  set_digital_output_params_at_switch_in=off  set_digital_outputs_at_start=on  set_digital_outputs_at_switch_in=off  set_digital_outputs_at_terminate=on  set_digital_outputs_at_switch_out=off  set_digital_outputs_on_watchdog=off  encoder_channels=[0:1]  quadrature=[4]  encoder_filter_frequency=[]  initial_encoder_counts=[0]  set_encoder_params_at_start=on  set_encoder_params_at_switch_in=off  set_encoder_counts_at_start=on  set_encoder_counts_at_switch_in=off  pwm_channels=[]  pwm_modes=[0]  pwm_frequency=1/0.020  pwm_configuration=[]  pwm_alignment=[]  pwm_polarity=[]  pwm_leading_deadband=[]  pwm_trailing_deadband=[]  initial_pwm_outputs=[0]  final_pwm_outputs=[0]  watchdog_pwm_outputs=[0]  set_pwm_params_at_start=on  set_pwm_params_at_switch_in=off  set_pwm_outputs_at_start=on  set_pwm_outputs_at_switch_in=off  set_pwm_outputs_at_terminate=on  set_pwm_outputs_at_switch_out=off  set_pwm_outputs_on_watchdog=off  other_output_channels=[]  initial_other_outputs=[]  final_other_outputs=[]  watchdog_other_outputs=[]  set_other_outputs_at_start=off  set_other_outputs_at_switch_in=off  set_other_outputs_at_terminate=off  set_other_outputs_at_switch_out=off  set_other_outputs_on_watchdog=off
  Mux : Mux  Inputs=2
  Voltage : quarc_library/Data Acquisition/Generic/Immediate I//O/HIL Write Analog  object_name=HIL-1  channels=0  sample_time=-1  active=off  vector_input=off
  counts to rad : Gain  Gain=2*pi/4096
  system out : Outport
  wires:
  sat control signal/1 -> Voltage/1
  Encoders/1 -> Gain/1
  Encoders/2 -> Mux/2
  Mux/1 -> counts to rad/1
  Gain/1 -> Mux/1
  counts to rad/1 -> system out/1

== system Controllers_Complete/Signal Builder1 ==
  Demux : Demux  Tag=STV Demux  Outputs=1
      settings: DisplayOption=none
  FromWs : FromWorkspace  Tag=STV FromWs  VariableName=tuvar
      SigBuilderData=|
      | common.afterFinalStr = 'Extrapolate'
      | common.sampleTime = 0
      | dataSet.timeRange = [0 10]
      | dataSet.name = 'Group 1'
      | sbobj.Groups.Name = 'Group 1'
      | sbobj.Groups.Signals.Name = 'Signal 1'
      | sbobj.Groups.Signals.XData = [0 1 1 3 3 5 5 7 7 8.5 8.5 10]
      | sbobj.Groups.Signals.YData = [0.005 0.005 40 40 15 15 -30 -30 0 0 23 23]
  Signal 1 : Outport  Tag=STV Outport
  wires:
  Demux/1 -> Signal 1/1
  FromWs/1 -> Demux/1

== system Controllers_Complete/State Extractor ==
  system out : Inport
  Demux7 : Demux  Outputs=2
  Derivative : Derivative
  Derivative1 : Derivative
  Mux2 : Mux
  Xhat : Outport
  wires:
  system out/1 -> Demux7/1
  Derivative1/1 -> Mux2/4  "alpha dot"
  Derivative/1 -> Mux2/2  "theta dot"
  Demux7/1 -> Mux2/1, Derivative/1  "theta"
  Demux7/2 -> Derivative1/1, Mux2/3  "alpha"
  Mux2/1 -> Xhat/1

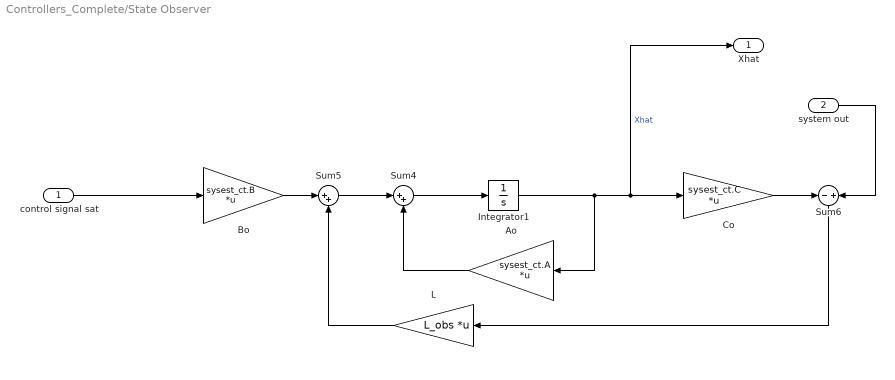
== system Controllers_Complete/State Observer ==
  control signal sat : Inport
  system out : Inport  Port=2
  Ao : Gain  Gain=sysest_ct.A  Multiplication=Matrix(K*u)
  Bo : Gain  Gain=sysest_ct.B  Multiplication=Matrix(K*u)
  Co : Gain  Gain=sysest_ct.C  Multiplication=Matrix(K*u)
  Integrator1 : Integrator
  L : Gain  Gain=L_obs  Multiplication=Matrix(K*u)
  Sum4 : Sum  Inputs=|++
  Sum5 : Sum  Inputs=|++
  Sum6 : Sum  Inputs=-+
  Xhat : Outport
  wires:
  system out/1 -> Sum6/2
  Ao/1 -> Sum4/2
  Sum4/1 -> Integrator1/1
  control signal sat/1 -> Bo/1
  Co/1 -> Sum6/1
  Sum6/1 -> L/1
  Bo/1 -> Sum5/1
  L/1 -> Sum5/2
  Integrator1/1 -> Xhat/1, Co/1, Ao/1  "Xhat"
  Sum5/1 -> Sum4/1

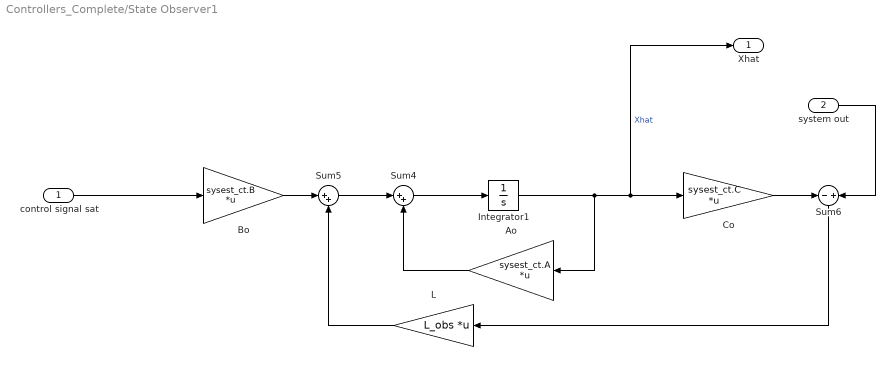
== system Controllers_Complete/State Observer1 ==
  control signal sat : Inport
  system out : Inport  Port=2
  Ao : Gain  Gain=sysest_ct.A  Multiplication=Matrix(K*u)
  Bo : Gain  Gain=sysest_ct.B  Multiplication=Matrix(K*u)
  Co : Gain  Gain=sysest_ct.C  Multiplication=Matrix(K*u)
  Integrator1 : Integrator
  L : Gain  Gain=L_obs  Multiplication=Matrix(K*u)
  Sum4 : Sum  Inputs=|++
  Sum5 : Sum  Inputs=|++
  Sum6 : Sum  Inputs=-+
  Xhat : Outport
  wires:
  system out/1 -> Sum6/2
  Ao/1 -> Sum4/2
  Sum4/1 -> Integrator1/1
  control signal sat/1 -> Bo/1
  Co/1 -> Sum6/1
  Sum6/1 -> L/1
  Bo/1 -> Sum5/1
  L/1 -> Sum5/2
  Integrator1/1 -> Xhat/1, Co/1, Ao/1  "Xhat"
  Sum5/1 -> Sum4/1

== system Controllers_Complete/fake ==
  sat control signal : Inport
  disturb : Inport  Port=2
  A1 : Gain  Gain=sysfake_ct.A  Multiplication=Matrix(K*u)
  B1 : Gain  Gain=sysfake_ct.B  Multiplication=Matrix(K*u)
  C1 : Gain  Gain=sysfake_ct.C  Multiplication=Matrix(K*u)
  Integrator2 : Integrator
  Sum7 : Sum  Inputs=|++
  Sum9 : Sum  Inputs=++|
  system out : Outport
  wires:
  Sum7/1 -> Integrator2/1
  disturb/1 -> Sum9/1
  B1/1 -> Sum7/1
  Integrator2/1 -> A1/1, C1/1  "xhat"
  C1/1 -> system out/1  "y"
  A1/1 -> Sum7/2
  sat control signal/1 -> Sum9/2
  Sum9/1 -> B1/1

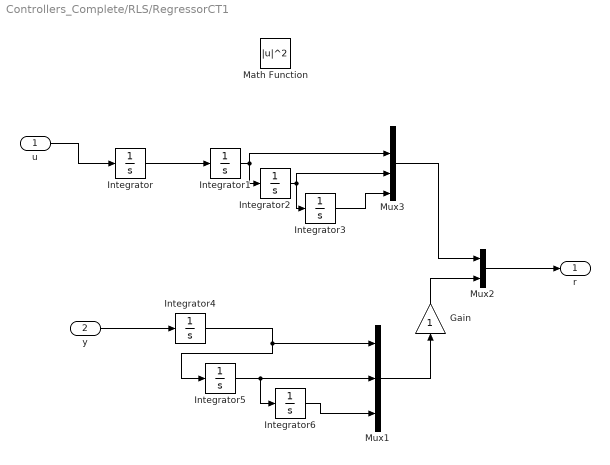
== system Controllers_Complete/RLS/RegressorCT1 ==
  u : Inport
  y : Inport  Port=2
  Gain : Gain
  Integrator{,1..6} (7 alike) : Integrator
  Math Function : Math  Operator=magnitude^2  SignedPower=on  SaturateOnIntegerOverflow=on
  Mux1 : Mux  Inputs=3
  Mux2 : Mux  Inputs=2
  Mux3 : Mux
  r : Outport  VectorParamsAs1DForOutWhenUnconnected=off
  wires:
  u/1 -> Integrator/1
  Mux2/1 -> r/1
  Integrator/1 -> Integrator1/1
  y/1 -> Integrator4/1
  Integrator4/1 -> Integrator5/1, Mux1/1
  Integrator1/1 -> Integrator2/1, Mux3/2
  Integrator2/1 -> Integrator3/1, Mux3/3
  Integrator3/1 -> Mux3/4
  Integrator5/1 -> Integrator6/1, Mux1/2
  Mux1/1 -> Gain/1
  Integrator6/1 -> Mux1/3
  Mux3/1 -> Mux2/1
  Gain/1 -> Mux2/2

== system Controllers_Complete/RLS/RegressorCTX1 ==
  Xhat : Inport
  Constant : Constant  Value=0
  Demux1 : Demux
  Integrator7 : Integrator
  Mux : Mux
  r : Outport  VectorParamsAs1DForOutWhenUnconnected=off
  wires:
  Xhat/1 -> Integrator7/1
  Demux1/2 -> Mux/2
  Integrator7/1 -> Demux1/1
  Demux1/3 -> Mux/3
  Demux1/4 -> Mux/4
  Mux/1 -> r/1
  Constant/1 -> Mux/1

== system Controllers_Complete/RLS/RegressorCTX2 ==
  Xhat : Inport
  Constant : Constant  Value=0
  Demux1 : Demux
  Integrator7 : Integrator
  Mux : Mux
  r : Outport  VectorParamsAs1DForOutWhenUnconnected=off
  wires:
  Xhat/1 -> Integrator7/1
  Demux1/2 -> Mux/2
  Integrator7/1 -> Demux1/1
  Demux1/3 -> Mux/3
  Demux1/4 -> Mux/4
  Mux/1 -> r/1
  Constant/1 -> Mux/1

== system Controllers_Complete/RLS/RegressorCTX3 ==
  Xhat : Inport
  Constant : Constant  Value=0
  Demux1 : Demux
  Integrator7 : Integrator
  Mux : Mux
  r : Outport  VectorParamsAs1DForOutWhenUnconnected=off
  wires:
  Xhat/1 -> Integrator7/1
  Integrator7/1 -> Demux1/1
  Demux1/4 -> Mux/4
  Mux/1 -> r/1
  Constant/1 -> Mux/3, Mux/2, Mux/1

== system Controllers_Complete/RLS/RegressorCTX4 ==
  Xhat : Inport
  Constant : Constant  Value=0
  Demux1 : Demux
  Integrator7 : Integrator
  Mux : Mux
  r : Outport  VectorParamsAs1DForOutWhenUnconnected=off
  wires:
  Xhat/1 -> Integrator7/1
  Integrator7/1 -> Demux1/1
  Demux1/4 -> Mux/4
  Mux/1 -> r/1
  Constant/1 -> Mux/1
  Demux1/2 -> Mux/2
  Demux1/3 -> Mux/3

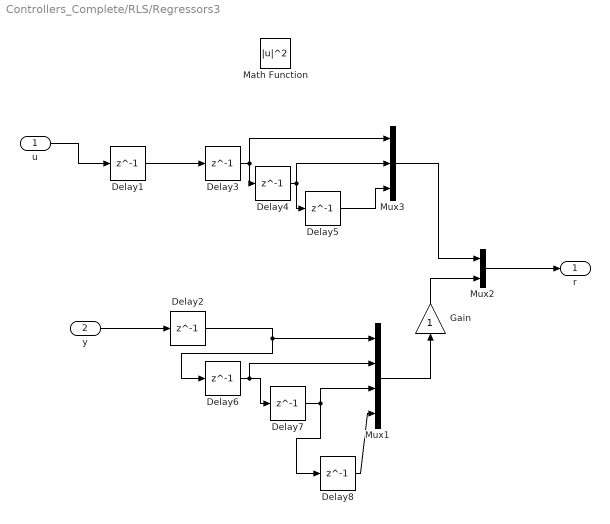
== system Controllers_Complete/RLS/Regressors3 ==
  u : Inport
  y : Inport  Port=2
  Delay{1..8} (8 alike) : Delay  DelayLength=1  InitialCondition=0  SampleTime=0.002
  Gain : Gain
  Math Function : Math  Operator=magnitude^2  SignedPower=on  SaturateOnIntegerOverflow=on
  Mux1 : Mux
  Mux2 : Mux  Inputs=2
  Mux3 : Mux  Inputs=3
  r : Outport  VectorParamsAs1DForOutWhenUnconnected=off
  wires:
  u/1 -> Delay1/1
  Mux2/1 -> r/1
  Delay1/1 -> Delay3/1
  y/1 -> Delay2/1
  Delay2/1 -> Mux1/1, Delay6/1
  Delay3/1 -> Mux3/1, Delay4/1
  Delay4/1 -> Mux3/2, Delay5/1
  Delay5/1 -> Mux3/3
  Delay6/1 -> Mux1/2, Delay7/1
  Mux1/1 -> Gain/1
  Delay7/1 -> Delay8/1, Mux1/3
  Delay8/1 -> Mux1/4
  Mux3/1 -> Mux2/1
  Gain/1 -> Mux2/2

== matlab function Controllers_Complete/Adaptive PP/MATLAB Function ==
  data: A input; K output; B input; pp_poles input; Kn output
function [K, Kn] = fcn(A,B,pp_poles)



Mr = [B, A*B, A*A*B, A*A*A*B];

pp_poles = pp_poles*-1;

a1 = pp_poles(1);
a2 = pp_poles(2);
a3 = pp_poles(3);
a4 = pp_poles(4);

p0 = a1*a2*a3*a4;
p1 = a1*a2*a3+  a1*a2*a4+   a1*a3*a4+   a2*a3*a4;
p2 = a1*a2+ a1*a3+ a1*a4+ a2*a3+ a2*a4+ a3*a4;
p3 = a1+a2+a3+a4;
p4 = 1;

PA = p4*A^4+ p3*A^3+ p2*A^2+ p1*A+ p0*eye(4);

K = [0 0 0 1]*inv(Mr)*PA;
kc = -[1 0 0 0; 0 0 1 0]*inv(A-B*K)*B;
Kn = 1/kc(1);

== matlab function Controllers_Complete/Kalman Filter Alp/MATLAB Function ==
  data: x_est input; y input; u input; x_est output; p_est input; p_est output; A input; B input; Q input; R input
function [x_est,p_est] = fcn(x_est,y,u,p_est, A,B,Q,R)
% Initialize state transition matrix
% Measurement matrix
H = [ 1 0 0 0; 0  0 1 0 ];


% Predicted state and covariance
x_prd = A * x_est + B* u;
p_prd = A * p_est * A' + Q;
% Estimation
S = p_prd'  + R;
B = p_prd';
klm_gain = (S \ B)';
% Estimated state and covariance
x_est = x_prd + klm_gain * (pinv(H)*y - x_prd);
p_est = p_prd - klm_gain  * p_prd;
% Compute the estimated measurements
end
